simulink model "PubIfDecisionTOS_MDL"  (R2020b)
settings: configuration reference "DspaceConfig" (kept outside this file)
PostLoadFcn:
  | if any(exist('dsrtsu_mdlpostloadfcn', 'file') ~= 0), dsrtsu_mdlpostloadfcn('Execute', bdroot); end
InitFcn:
  | , if any(exist('dsmpb_private', 'file') ~= 0), dsmpb_private('dsmpb_mdlclblib', 'Init', bdroot); end,
undefined symbols (not defined in the file or in its folder): C_TOS_ACCEgoRAxletoFbumplength_m, C_TOS_ACCTargetFront_Flag, C_TOS_AEBJAPedObjDxThre_Val, C_TOS_AEBJAPedObjDyThre_Val, C_TOS_AEBJATargetSize_Val, C_TOS_AEBJAVehObjDxThre_Val, C_TOS_AEBJAVehObjDyThre_Val, C_TOS_AEBJuncPedTargetSize_Val, C_TOS_AEBLatObjDxThre_Val, C_TOS_AEBLatPedDyThre_Val, C_TOS_AEBLatTargetSize_Val, C_TOS_AEBLongTargetInEgoFront_Flag, C_TOS_axAbsGround_Parameter, C_TOS_CameraConfirmedFlag, C_TOS_CNsubjWidth, C_TOS_CurrentLaneCoreMinWidth_Val, C_TOS_CutInProb_Val_Zero, C_TOS_CutOutProb_Val_Zero, C_TOS_D2R_Val, C_TOS_DefaultValueObjectToCenterLine_dy, C_TOS_EgoCarWidth_Val, C_TOS_EgoDxRefPoint_m, C_TOS_EgoRAxletoFbumplength_m, C_TOS_HalfWidthVehicle_Con, C_TOS_HWA_CurrentLaneFlag, C_TOS_HWA_LeftLaneFlag, C_TOS_HWA_MovingDir_Vaild, C_TOS_HWA_MovState_Vaild, C_TOS_HWA_RightLaneFlag, C_TOS_LaneLineCourseErrorFront, C_TOS_LaneLineCourseErrorRear, C_TOS_MotorbikeDefaultWidth_m, C_TOS_NumberOfEffectiveTargets, C_TOS_Obj_Age_Val, C_TOS_Objdx_Constraint_Val, C_TOS_ObjectDefaultWidth_m, C_TOS_ObjInCurrentLane_Val, C_TOS_ObjInCurrentLaneValid, C_TOS_ObjInLeftLaneValid, C_TOS_ObjInRightLaneValid, C_TOS_ObjNotInCurrentLane_Val, C_TOS_ObjNotREElementType, C_TOS_ObjPredictDis_dy_ConstantVal_Zeros, C_TOS_ObjToCenterLine_ConstantVal_Zeros, C_TOS_OFMObjIDInvilad_Val, C_TOS_PIL_LatDisCons_Val_zero, C_TOS_PIL_ObjectCutInFlag_b, C_TOS_PIL_ObjectCutOutFlag_b, C_TOS_PIL_ObjLaneProb_al_Val, C_TOS_PP_ObjFusType_FC_Confirm_b, C_TOS_PP_ObjFusType_FC_FR_Confirm_b, C_TOS_PP_ObjFusType_FR_Confirm_b, C_TOS_RE_80BoolDefault_Val, C_TOS_RE_80Single181Default_Val, C_TOS_RE_80Single255Default_Val, C_TOS_RE_80Uint8Default_Val, C_TOS_RE_D2R, C_TOS_RE_D_180_Val, C_TOS_RE_InvalidObjectID_Val, C_TOS_RE_InvalidTargetChainDir_Val ... (+142)
libraries: simulink x1650, TOS_LIB x361, canfdmsglib x14
(part 10 of 69)

== system PubIfDecisionTOS_MDL/TOS_20201112/TOS_2012080320/PIL_1029/ProbCalculat/ProbFilt/ObjinLeftLaneProb ==
  PIL_ObjinLeftLaneProb : Inport
  Demux : Demux  Outputs=80
  Mux : Mux  Inputs=80
  Prob_Filt{1..80} (80 alike) : TOS_LIB/Prob_Filt  SystemSampleTime=-1  VariantActivationTime=update diagram  Latency=0  AutoFrameSizeCalculation=off
  PIL_ObjinLeftLaneProb_Filt : Outport
  wires:
  PIL_ObjinLeftLaneProb/1 -> Demux/1
  Demux/1 -> Prob_Filt1/1
  Demux/80 -> Prob_Filt72/1
  Demux/79 -> Prob_Filt71/1
  Demux/78 -> Prob_Filt70/1
  Demux/77 -> Prob_Filt69/1
  Demux/76 -> Prob_Filt68/1
  Demux/75 -> Prob_Filt67/1
  Demux/74 -> Prob_Filt66/1
  Demux/73 -> Prob_Filt80/1
  Demux/72 -> Prob_Filt79/1
  Demux/71 -> Prob_Filt78/1
  Demux/70 -> Prob_Filt77/1
  Demux/69 -> Prob_Filt76/1
  Demux/68 -> Prob_Filt75/1
  Demux/61 -> Prob_Filt46/1
  Demux/2 -> Prob_Filt2/1
  Demux/3 -> Prob_Filt3/1
  Demux/4 -> Prob_Filt4/1
  Demux/5 -> Prob_Filt5/1
  Demux/6 -> Prob_Filt6/1
  Demux/7 -> Prob_Filt7/1
  Demux/8 -> Prob_Filt8/1
  Demux/9 -> Prob_Filt9/1
  Demux/10 -> Prob_Filt10/1
  Demux/11 -> Prob_Filt11/1
  Demux/12 -> Prob_Filt12/1
  Demux/13 -> Prob_Filt13/1
  Demux/14 -> Prob_Filt14/1
  Demux/15 -> Prob_Filt15/1
  Demux/16 -> Prob_Filt16/1
  Demux/17 -> Prob_Filt17/1
  Demux/18 -> Prob_Filt25/1
  Demux/19 -> Prob_Filt26/1
  Demux/20 -> Prob_Filt27/1
  Demux/21 -> Prob_Filt28/1
  Demux/22 -> Prob_Filt29/1
  Demux/23 -> Prob_Filt30/1
  Demux/24 -> Prob_Filt31/1
  Demux/25 -> Prob_Filt32/1
  Demux/26 -> Prob_Filt18/1
  Demux/27 -> Prob_Filt19/1
  Demux/28 -> Prob_Filt20/1
  Demux/29 -> Prob_Filt21/1
  Demux/30 -> Prob_Filt22/1
  Demux/31 -> Prob_Filt23/1
  Demux/32 -> Prob_Filt24/1
  Demux/33 -> Prob_Filt33/1
  Demux/34 -> Prob_Filt44/1
  Demux/35 -> Prob_Filt55/1
  Demux/36 -> Prob_Filt59/1
  Demux/37 -> Prob_Filt60/1
  Demux/38 -> Prob_Filt61/1
  Demux/39 -> Prob_Filt62/1
  Demux/40 -> Prob_Filt63/1
  Demux/41 -> Prob_Filt64/1
  Demux/42 -> Prob_Filt34/1
  Demux/43 -> Prob_Filt35/1
  Demux/44 -> Prob_Filt36/1
  Demux/45 -> Prob_Filt37/1
  Demux/46 -> Prob_Filt38/1
  Demux/47 -> Prob_Filt39/1
  Demux/48 -> Prob_Filt40/1
  Demux/49 -> Prob_Filt41/1
  Demux/50 -> Prob_Filt50/1
  Demux/51 -> Prob_Filt51/1
  Demux/52 -> Prob_Filt52/1
  Demux/53 -> Prob_Filt53/1
  Demux/54 -> Prob_Filt54/1
  Demux/55 -> Prob_Filt56/1
  Demux/56 -> Prob_Filt57/1
  Demux/57 -> Prob_Filt58/1
  Demux/58 -> Prob_Filt42/1
  Demux/59 -> Prob_Filt43/1
  Demux/60 -> Prob_Filt45/1
  Demux/62 -> Prob_Filt47/1
  Demux/63 -> Prob_Filt48/1
  Demux/64 -> Prob_Filt49/1
  Demux/65 -> Prob_Filt65/1
  Demux/66 -> Prob_Filt73/1
  Demux/67 -> Prob_Filt74/1
  Prob_Filt1/1 -> Mux/1  "EgoCar_LeftLaneProb"
  Prob_Filt2/1 -> Mux/2  "EgoCar_LeftLaneProb"
  Prob_Filt3/1 -> Mux/3  "EgoCar_LeftLaneProb"
  Prob_Filt4/1 -> Mux/4  "EgoCar_LeftLaneProb"
  Prob_Filt5/1 -> Mux/5  "EgoCar_LeftLaneProb"
  Prob_Filt6/1 -> Mux/6  "EgoCar_LeftLaneProb"
  Prob_Filt7/1 -> Mux/7  "EgoCar_LeftLaneProb"
  Prob_Filt8/1 -> Mux/8  "EgoCar_LeftLaneProb"
  Prob_Filt9/1 -> Mux/9  "EgoCar_LeftLaneProb"
  Prob_Filt10/1 -> Mux/10  "EgoCar_LeftLaneProb"
  Prob_Filt11/1 -> Mux/11  "EgoCar_LeftLaneProb"
  Prob_Filt12/1 -> Mux/12  "EgoCar_LeftLaneProb"
  Prob_Filt13/1 -> Mux/13  "EgoCar_LeftLaneProb"
  Prob_Filt14/1 -> Mux/14  "EgoCar_LeftLaneProb"
  Prob_Filt15/1 -> Mux/15  "EgoCar_LeftLaneProb"
  Prob_Filt16/1 -> Mux/16  "EgoCar_LeftLaneProb"
  Prob_Filt17/1 -> Mux/17  "EgoCar_LeftLaneProb"
  Prob_Filt25/1 -> Mux/18  "EgoCar_LeftLaneProb"
  Prob_Filt26/1 -> Mux/19  "EgoCar_LeftLaneProb"
  Prob_Filt27/1 -> Mux/20  "EgoCar_LeftLaneProb"
  Prob_Filt28/1 -> Mux/21  "EgoCar_LeftLaneProb"
  Prob_Filt29/1 -> Mux/22  "EgoCar_LeftLaneProb"
  Prob_Filt30/1 -> Mux/23  "EgoCar_LeftLaneProb"
  Prob_Filt31/1 -> Mux/24  "EgoCar_LeftLaneProb"
  Prob_Filt32/1 -> Mux/25  "EgoCar_LeftLaneProb"
  Prob_Filt18/1 -> Mux/26  "EgoCar_LeftLaneProb"
  Prob_Filt19/1 -> Mux/27  "EgoCar_LeftLaneProb"
  Prob_Filt20/1 -> Mux/28  "EgoCar_LeftLaneProb"
  Prob_Filt21/1 -> Mux/29  "EgoCar_LeftLaneProb"
  Prob_Filt22/1 -> Mux/30  "EgoCar_LeftLaneProb"
  Prob_Filt23/1 -> Mux/31  "EgoCar_LeftLaneProb"
  Prob_Filt24/1 -> Mux/32  "EgoCar_LeftLaneProb"
  Prob_Filt33/1 -> Mux/33  "EgoCar_LeftLaneProb"
  Prob_Filt44/1 -> Mux/34  "EgoCar_LeftLaneProb"
  Prob_Filt55/1 -> Mux/35  "EgoCar_LeftLaneProb"
  Prob_Filt59/1 -> Mux/36  "EgoCar_LeftLaneProb"
  Prob_Filt60/1 -> Mux/37  "EgoCar_LeftLaneProb"
  Prob_Filt61/1 -> Mux/38  "EgoCar_LeftLaneProb"
  Prob_Filt62/1 -> Mux/39  "EgoCar_LeftLaneProb"
  Prob_Filt63/1 -> Mux/40  "EgoCar_LeftLaneProb"
  Prob_Filt64/1 -> Mux/41  "EgoCar_LeftLaneProb"
  Prob_Filt34/1 -> Mux/42  "EgoCar_LeftLaneProb"
  Prob_Filt35/1 -> Mux/43  "EgoCar_LeftLaneProb"
  Prob_Filt36/1 -> Mux/44  "EgoCar_LeftLaneProb"
  Prob_Filt37/1 -> Mux/45  "EgoCar_LeftLaneProb"
  Prob_Filt38/1 -> Mux/46  "EgoCar_LeftLaneProb"
  Prob_Filt39/1 -> Mux/47  "EgoCar_LeftLaneProb"
  Prob_Filt40/1 -> Mux/48  "EgoCar_LeftLaneProb"
  Prob_Filt41/1 -> Mux/49  "EgoCar_LeftLaneProb"
  Prob_Filt50/1 -> Mux/50  "EgoCar_LeftLaneProb"
  Prob_Filt51/1 -> Mux/51  "EgoCar_LeftLaneProb"
  Prob_Filt52/1 -> Mux/52  "EgoCar_LeftLaneProb"
  Prob_Filt53/1 -> Mux/53  "EgoCar_LeftLaneProb"
  Prob_Filt54/1 -> Mux/54  "EgoCar_LeftLaneProb"
  Prob_Filt56/1 -> Mux/55  "EgoCar_LeftLaneProb"
  Prob_Filt57/1 -> Mux/56  "EgoCar_LeftLaneProb"
  Prob_Filt58/1 -> Mux/57  "EgoCar_LeftLaneProb"
  Prob_Filt42/1 -> Mux/58  "EgoCar_LeftLaneProb"
  Prob_Filt43/1 -> Mux/59  "EgoCar_LeftLaneProb"
  Prob_Filt45/1 -> Mux/60  "EgoCar_LeftLaneProb"
  Prob_Filt46/1 -> Mux/61  "EgoCar_LeftLaneProb"
  Prob_Filt47/1 -> Mux/62  "EgoCar_LeftLaneProb"
  Prob_Filt48/1 -> Mux/63  "EgoCar_LeftLaneProb"
  Prob_Filt49/1 -> Mux/64  "EgoCar_LeftLaneProb"
  Prob_Filt65/1 -> Mux/65  "EgoCar_LeftLaneProb"
  Prob_Filt73/1 -> Mux/66  "EgoCar_LeftLaneProb"
  Prob_Filt74/1 -> Mux/67  "EgoCar_LeftLaneProb"
  Prob_Filt75/1 -> Mux/68  "EgoCar_LeftLaneProb"
  Prob_Filt76/1 -> Mux/69  "EgoCar_LeftLaneProb"
  Prob_Filt77/1 -> Mux/70  "EgoCar_LeftLaneProb"
  Prob_Filt78/1 -> Mux/71  "EgoCar_LeftLaneProb"
  Prob_Filt79/1 -> Mux/72  "EgoCar_LeftLaneProb"
  Prob_Filt80/1 -> Mux/73  "EgoCar_LeftLaneProb"
  Prob_Filt66/1 -> Mux/74  "EgoCar_LeftLaneProb"
  Prob_Filt67/1 -> Mux/75  "EgoCar_LeftLaneProb"
  Prob_Filt68/1 -> Mux/76  "EgoCar_LeftLaneProb"
  Prob_Filt69/1 -> Mux/77  "EgoCar_LeftLaneProb"
  Prob_Filt70/1 -> Mux/78  "EgoCar_LeftLaneProb"
  Prob_Filt71/1 -> Mux/79  "EgoCar_LeftLaneProb"
  Prob_Filt72/1 -> Mux/80  "EgoCar_LeftLaneProb"
  Mux/1 -> PIL_ObjinLeftLaneProb_Filt/1

== system PubIfDecisionTOS_MDL/TOS_20201112/TOS_2012080320/PIL_1029/ProbCalculat/ProbFilt/ObjinRightLaneProb ==
  PIL_ObjinRightLaneProb : Inport
  Demux : Demux  Outputs=80
  Mux : Mux  Inputs=80
  Prob_Filt{1..80} (80 alike) : TOS_LIB/Prob_Filt  SystemSampleTime=-1  VariantActivationTime=update diagram  Latency=0  AutoFrameSizeCalculation=off
  PIL_ObjinRightLaneProb_Filt : Outport
  wires:
  PIL_ObjinRightLaneProb/1 -> Demux/1
  Demux/1 -> Prob_Filt1/1
  Demux/80 -> Prob_Filt72/1
  Demux/79 -> Prob_Filt71/1
  Demux/78 -> Prob_Filt70/1
  Demux/77 -> Prob_Filt69/1
  Demux/76 -> Prob_Filt68/1
  Demux/75 -> Prob_Filt67/1
  Demux/74 -> Prob_Filt66/1
  Demux/73 -> Prob_Filt80/1
  Demux/72 -> Prob_Filt79/1
  Demux/71 -> Prob_Filt78/1
  Demux/70 -> Prob_Filt77/1
  Demux/69 -> Prob_Filt76/1
  Demux/68 -> Prob_Filt75/1
  Demux/61 -> Prob_Filt46/1
  Demux/2 -> Prob_Filt2/1
  Demux/3 -> Prob_Filt3/1
  Demux/4 -> Prob_Filt4/1
  Demux/5 -> Prob_Filt5/1
  Demux/6 -> Prob_Filt6/1
  Demux/7 -> Prob_Filt7/1
  Demux/8 -> Prob_Filt8/1
  Demux/9 -> Prob_Filt9/1
  Demux/10 -> Prob_Filt10/1
  Demux/11 -> Prob_Filt11/1
  Demux/12 -> Prob_Filt12/1
  Demux/13 -> Prob_Filt13/1
  Demux/14 -> Prob_Filt14/1
  Demux/15 -> Prob_Filt15/1
  Demux/16 -> Prob_Filt16/1
  Demux/17 -> Prob_Filt17/1
  Demux/18 -> Prob_Filt25/1
  Demux/19 -> Prob_Filt26/1
  Demux/20 -> Prob_Filt27/1
  Demux/21 -> Prob_Filt28/1
  Demux/22 -> Prob_Filt29/1
  Demux/23 -> Prob_Filt30/1
  Demux/24 -> Prob_Filt31/1
  Demux/25 -> Prob_Filt32/1
  Demux/26 -> Prob_Filt18/1
  Demux/27 -> Prob_Filt19/1
  Demux/28 -> Prob_Filt20/1
  Demux/29 -> Prob_Filt21/1
  Demux/30 -> Prob_Filt22/1
  Demux/31 -> Prob_Filt23/1
  Demux/32 -> Prob_Filt24/1
  Demux/33 -> Prob_Filt33/1
  Demux/34 -> Prob_Filt44/1
  Demux/35 -> Prob_Filt55/1
  Demux/36 -> Prob_Filt59/1
  Demux/37 -> Prob_Filt60/1
  Demux/38 -> Prob_Filt61/1
  Demux/39 -> Prob_Filt62/1
  Demux/40 -> Prob_Filt63/1
  Demux/41 -> Prob_Filt64/1
  Demux/42 -> Prob_Filt34/1
  Demux/43 -> Prob_Filt35/1
  Demux/44 -> Prob_Filt36/1
  Demux/45 -> Prob_Filt37/1
  Demux/46 -> Prob_Filt38/1
  Demux/47 -> Prob_Filt39/1
  Demux/48 -> Prob_Filt40/1
  Demux/49 -> Prob_Filt41/1
  Demux/50 -> Prob_Filt50/1
  Demux/51 -> Prob_Filt51/1
  Demux/52 -> Prob_Filt52/1
  Demux/53 -> Prob_Filt53/1
  Demux/54 -> Prob_Filt54/1
  Demux/55 -> Prob_Filt56/1
  Demux/56 -> Prob_Filt57/1
  Demux/57 -> Prob_Filt58/1
  Demux/58 -> Prob_Filt42/1
  Demux/59 -> Prob_Filt43/1
  Demux/60 -> Prob_Filt45/1
  Demux/62 -> Prob_Filt47/1
  Demux/63 -> Prob_Filt48/1
  Demux/64 -> Prob_Filt49/1
  Demux/65 -> Prob_Filt65/1
  Demux/66 -> Prob_Filt73/1
  Demux/67 -> Prob_Filt74/1
  Prob_Filt1/1 -> Mux/1  "EgoCar_LeftLaneProb"
  Prob_Filt2/1 -> Mux/2  "EgoCar_LeftLaneProb"
  Prob_Filt3/1 -> Mux/3  "EgoCar_LeftLaneProb"
  Prob_Filt4/1 -> Mux/4  "EgoCar_LeftLaneProb"
  Prob_Filt5/1 -> Mux/5  "EgoCar_LeftLaneProb"
  Prob_Filt6/1 -> Mux/6  "EgoCar_LeftLaneProb"
  Prob_Filt7/1 -> Mux/7  "EgoCar_LeftLaneProb"
  Prob_Filt8/1 -> Mux/8  "EgoCar_LeftLaneProb"
  Prob_Filt9/1 -> Mux/9  "EgoCar_LeftLaneProb"
  Prob_Filt10/1 -> Mux/10  "EgoCar_LeftLaneProb"
  Prob_Filt11/1 -> Mux/11  "EgoCar_LeftLaneProb"
  Prob_Filt12/1 -> Mux/12  "EgoCar_LeftLaneProb"
  Prob_Filt13/1 -> Mux/13  "EgoCar_LeftLaneProb"
  Prob_Filt14/1 -> Mux/14  "EgoCar_LeftLaneProb"
  Prob_Filt15/1 -> Mux/15  "EgoCar_LeftLaneProb"
  Prob_Filt16/1 -> Mux/16  "EgoCar_LeftLaneProb"
  Prob_Filt17/1 -> Mux/17  "EgoCar_LeftLaneProb"
  Prob_Filt25/1 -> Mux/18  "EgoCar_LeftLaneProb"
  Prob_Filt26/1 -> Mux/19  "EgoCar_LeftLaneProb"
  Prob_Filt27/1 -> Mux/20  "EgoCar_LeftLaneProb"
  Prob_Filt28/1 -> Mux/21  "EgoCar_LeftLaneProb"
  Prob_Filt29/1 -> Mux/22  "EgoCar_LeftLaneProb"
  Prob_Filt30/1 -> Mux/23  "EgoCar_LeftLaneProb"
  Prob_Filt31/1 -> Mux/24  "EgoCar_LeftLaneProb"
  Prob_Filt32/1 -> Mux/25  "EgoCar_LeftLaneProb"
  Prob_Filt18/1 -> Mux/26  "EgoCar_LeftLaneProb"
  Prob_Filt19/1 -> Mux/27  "EgoCar_LeftLaneProb"
  Prob_Filt20/1 -> Mux/28  "EgoCar_LeftLaneProb"
  Prob_Filt21/1 -> Mux/29  "EgoCar_LeftLaneProb"
  Prob_Filt22/1 -> Mux/30  "EgoCar_LeftLaneProb"
  Prob_Filt23/1 -> Mux/31  "EgoCar_LeftLaneProb"
  Prob_Filt24/1 -> Mux/32  "EgoCar_LeftLaneProb"
  Prob_Filt33/1 -> Mux/33  "EgoCar_LeftLaneProb"
  Prob_Filt44/1 -> Mux/34  "EgoCar_LeftLaneProb"
  Prob_Filt55/1 -> Mux/35  "EgoCar_LeftLaneProb"
  Prob_Filt59/1 -> Mux/36  "EgoCar_LeftLaneProb"
  Prob_Filt60/1 -> Mux/37  "EgoCar_LeftLaneProb"
  Prob_Filt61/1 -> Mux/38  "EgoCar_LeftLaneProb"
  Prob_Filt62/1 -> Mux/39  "EgoCar_LeftLaneProb"
  Prob_Filt63/1 -> Mux/40  "EgoCar_LeftLaneProb"
  Prob_Filt64/1 -> Mux/41  "EgoCar_LeftLaneProb"
  Prob_Filt34/1 -> Mux/42  "EgoCar_LeftLaneProb"
  Prob_Filt35/1 -> Mux/43  "EgoCar_LeftLaneProb"
  Prob_Filt36/1 -> Mux/44  "EgoCar_LeftLaneProb"
  Prob_Filt37/1 -> Mux/45  "EgoCar_LeftLaneProb"
  Prob_Filt38/1 -> Mux/46  "EgoCar_LeftLaneProb"
  Prob_Filt39/1 -> Mux/47  "EgoCar_LeftLaneProb"
  Prob_Filt40/1 -> Mux/48  "EgoCar_LeftLaneProb"
  Prob_Filt41/1 -> Mux/49  "EgoCar_LeftLaneProb"
  Prob_Filt50/1 -> Mux/50  "EgoCar_LeftLaneProb"
  Prob_Filt51/1 -> Mux/51  "EgoCar_LeftLaneProb"
  Prob_Filt52/1 -> Mux/52  "EgoCar_LeftLaneProb"
  Prob_Filt53/1 -> Mux/53  "EgoCar_LeftLaneProb"
  Prob_Filt54/1 -> Mux/54  "EgoCar_LeftLaneProb"
  Prob_Filt56/1 -> Mux/55  "EgoCar_LeftLaneProb"
  Prob_Filt57/1 -> Mux/56  "EgoCar_LeftLaneProb"
  Prob_Filt58/1 -> Mux/57  "EgoCar_LeftLaneProb"
  Prob_Filt42/1 -> Mux/58  "EgoCar_LeftLaneProb"
  Prob_Filt43/1 -> Mux/59  "EgoCar_LeftLaneProb"
  Prob_Filt45/1 -> Mux/60  "EgoCar_LeftLaneProb"
  Prob_Filt46/1 -> Mux/61  "EgoCar_LeftLaneProb"
  Prob_Filt47/1 -> Mux/62  "EgoCar_LeftLaneProb"
  Prob_Filt48/1 -> Mux/63  "EgoCar_LeftLaneProb"
  Prob_Filt49/1 -> Mux/64  "EgoCar_LeftLaneProb"
  Prob_Filt65/1 -> Mux/65  "EgoCar_LeftLaneProb"
  Prob_Filt73/1 -> Mux/66  "EgoCar_LeftLaneProb"
  Prob_Filt74/1 -> Mux/67  "EgoCar_LeftLaneProb"
  Prob_Filt75/1 -> Mux/68  "EgoCar_LeftLaneProb"
  Prob_Filt76/1 -> Mux/69  "EgoCar_LeftLaneProb"
  Prob_Filt77/1 -> Mux/70  "EgoCar_LeftLaneProb"
  Prob_Filt78/1 -> Mux/71  "EgoCar_LeftLaneProb"
  Prob_Filt79/1 -> Mux/72  "EgoCar_LeftLaneProb"
  Prob_Filt80/1 -> Mux/73  "EgoCar_LeftLaneProb"
  Prob_Filt66/1 -> Mux/74  "EgoCar_LeftLaneProb"
  Prob_Filt67/1 -> Mux/75  "EgoCar_LeftLaneProb"
  Prob_Filt68/1 -> Mux/76  "EgoCar_LeftLaneProb"
  Prob_Filt69/1 -> Mux/77  "EgoCar_LeftLaneProb"
  Prob_Filt70/1 -> Mux/78  "EgoCar_LeftLaneProb"
  Prob_Filt71/1 -> Mux/79  "EgoCar_LeftLaneProb"
  Prob_Filt72/1 -> Mux/80  "EgoCar_LeftLaneProb"
  Mux/1 -> PIL_ObjinRightLaneProb_Filt/1

== system PubIfDecisionTOS_MDL/TOS_20201112/TOS_2012080320/PP1128/AAT-AdditionalAttributes/PP_CenterLine_Calculat/EgoLane_CenterLine ==
  EgoLane : Inport
  Bus Creator1 : BusCreator  Inputs=6
  EgoLaneCenterLine01 : Subsystem
  EgoLaneCenterLine02 : Subsystem
  EgoLaneCenterLine03 : Subsystem
  EgoLaneCenterLine04 : Subsystem
  EgoLaneCenterLine05 : Subsystem
  EgoLaneCenterLine06 : Subsystem
  PP_EgoLane_CenterLine : Outport
  wires:
  EgoLane/1 -> EgoLaneCenterLine03/1(EgoLaneLine), EgoLaneCenterLine06/1(EgoLaneLine), EgoLaneCenterLine05/1(EgoLaneLine), EgoLaneCenterLine04/1(EgoLaneLine), EgoLaneCenterLine02/1(EgoLaneLine), EgoLaneCenterLine01/1(EgoLaneLine)
  EgoLaneCenterLine01/1(EgoLaneCenterLine01) -> Bus Creator1/1  "CenterLine01"
  EgoLaneCenterLine06/1(EgoLaneCenterLine06) -> Bus Creator1/6  "CenterLine06"
  EgoLaneCenterLine02/1(EgoLaneCenterLine02) -> Bus Creator1/2  "CenterLine02"
  EgoLaneCenterLine03/1(EgoLaneCenterLine03) -> Bus Creator1/3  "CenterLine03"
  EgoLaneCenterLine04/1(EgoLaneCenterLine04) -> Bus Creator1/4  "CenterLine04"
  EgoLaneCenterLine05/1(EgoLaneCenterLine05) -> Bus Creator1/5  "CenterLine05"
  Bus Creator1/1 -> PP_EgoLane_CenterLine/1  "PP_EgoLane_CenterLine"

== system PubIfDecisionTOS_MDL/TOS_20201112/TOS_2012080320/PP1128/AAT-AdditionalAttributes/PP_CenterLine_Calculat/LaneWidth ==
  LM_SignalVerification : Inport
  Add : Sum  Inputs=+-  OutDataTypeStr=single
  Add1 : Sum  Inputs=+-  OutDataTypeStr=single
  Add2 : Sum  Inputs=+-  OutDataTypeStr=single
  Bus Creator : BusCreator  Inputs=3
  Bus Selector1 : BusSelector  OutputSignals=TOS_LM_LL_Bus.LM_LL_Line04.pC0,TOS_LM_LR_Bus.LM_LR_Line04.pC0,TOS_LM_RL_Bus.LM_RL_Line04.pC0,TOS_LM_RR_Bus.LM_RR_Line04.pC0
  Saturation : Saturate  UpperLimit=4  LowerLimit=2.0  OutDataTypeStr=single
  Saturation1 : Saturate  UpperLimit=4  LowerLimit=2.0  OutDataTypeStr=single
  Saturation2 : Saturate  UpperLimit=4  LowerLimit=2.0  OutDataTypeStr=single
  Signal Copy{,1..3} (4 alike) : SignalConversion  OverrideOpt=off
  Subsystem : Subsystem  Commented=on
  PP_LaneWidth : Outport
  wires:
  Saturation/1 -> Bus Creator/1  "TOS_PP_LeftLaneWidth"
  LM_SignalVerification/1 -> Bus Selector1/1
  Saturation1/1 -> Bus Creator/2  "TOS_PP_CurrentLaneWidth"
  Bus Creator/1 -> PP_LaneWidth/1
  Saturation2/1 -> Bus Creator/3  "TOS_PP_RightLaneWidth"
  Bus Selector1/4 -> Signal Copy3/1  "<pC0>"
  Signal Copy/1 -> Add/1  "LM_LL_pC0"
  Signal Copy3/1 -> Add2/2  "LM_RR_pC0"
  Bus Selector1/2 -> Signal Copy1/1  "<pC0>"
  Add/1 -> Saturation/1
  Signal Copy1/1 -> Add1/1, Add/2  "LM_LR_pC0"
  Add1/1 -> Saturation1/1
  Bus Selector1/3 -> Signal Copy2/1  "<pC0>"
  Signal Copy2/1 -> Add1/2, Add2/1  "LM_RL_pC0"
  Add2/1 -> Saturation2/1
  Bus Selector1/1 -> Signal Copy/1  "<pC0>"

== system PubIfDecisionTOS_MDL/TOS_20201112/TOS_2012080320/PP1128/AAT-AdditionalAttributes/PP_CenterLine_Calculat/LaneWidth_80 ==
  OFM_SignalVerification : Inport
  LM_SignalVerification : Inport  Port=2
  Bus Creator : BusCreator  Inputs=3
  Bus Selector : BusSelector  OutputSignals=TOS_OFMObjValid_Flag,Object_MovingState,Object_Type
  Bus Selector1 : BusSelector  OutputSignals=TOS_LM_LL_Bus.LM_LL_Line04.pC0,TOS_LM_LR_Bus.LM_LR_Line04.pC0,TOS_LM_RL_Bus.LM_RL_Line04.pC0,TOS_LM_RR_Bus.LM_RR_Line04.pC0
  LaneWidth : Subsystem
  PP_LaneWidth : Outport
  wires:
  Bus Selector1/4 -> LaneWidth/7(LM_RR_pC0)  "<pC0>"
  Bus Selector1/3 -> LaneWidth/6(LM_RL_pC0)  "<pC0>"
  Bus Selector1/2 -> LaneWidth/5(LM_LR_pC0)  "<pC0>"
  Bus Selector1/1 -> LaneWidth/4(LM_LL_pC0)  "<pC0>"
  LaneWidth/3(TOS_PP_RightLaneWidth) -> Bus Creator/3  "TOS_PP_RightLaneWidth"
  Bus Creator/1 -> PP_LaneWidth/1
  LaneWidth/1(TOS_PP_CurrentLaneWidth) -> Bus Creator/1  "TOS_PP_CurrentLaneWidth"
  LM_SignalVerification/1 -> Bus Selector1/1
  Bus Selector/2 -> LaneWidth/2(Object_MovingState)  "<Object_MovingState>"
  Bus Selector/1 -> LaneWidth/1(TOS_OFMObjValid_Flag)  "<TOS_OFMObjValid_Flag>"
  Bus Selector/3 -> LaneWidth/3(Object_Type)  "<Object_Type>"
  OFM_SignalVerification/1 -> Bus Selector/1
  LaneWidth/2(TOS_PP_LeftLaneWidth) -> Bus Creator/2  "TOS_PP_LeftLaneWidth"

== system PubIfDecisionTOS_MDL/TOS_20201112/TOS_2012080320/PP1128/AAT-AdditionalAttributes/PP_CenterLine_Calculat/LeftLane_CenterLine ==
  LeftLane : Inport
  Bus Creator1 : BusCreator  Inputs=6
  LaneCenterLine01 : Subsystem
  LaneCenterLine02 : Subsystem
  LaneCenterLine03 : Subsystem
  LaneCenterLine04 : Subsystem
  LaneCenterLine05 : Subsystem
  LaneCenterLine06 : Subsystem
  PP_LeftLane_CenterLine : Outport
  wires:
  LeftLane/1 -> LaneCenterLine01/1(LaneLine), LaneCenterLine02/1(LaneLine), LaneCenterLine03/1(LaneLine), LaneCenterLine04/1(LaneLine), LaneCenterLine05/1(LaneLine), LaneCenterLine06/1(LaneLine)
  LaneCenterLine01/1(LaneCenterLine01) -> Bus Creator1/1  "CenterLine01"
  LaneCenterLine06/1(LaneCenterLine06) -> Bus Creator1/6  "CenterLine06"
  LaneCenterLine02/1(LaneCenterLine02) -> Bus Creator1/2  "CenterLine02"
  LaneCenterLine03/1(LaneCenterLine03) -> Bus Creator1/3  "CenterLine03"
  LaneCenterLine04/1(LaneCenterLine04) -> Bus Creator1/4  "CenterLine04"
  LaneCenterLine05/1(LaneCenterLine05) -> Bus Creator1/5  "CenterLine05"
  Bus Creator1/1 -> PP_LeftLane_CenterLine/1  "PP_LeftLane_CenterLine"

== system PubIfDecisionTOS_MDL/TOS_20201112/TOS_2012080320/PP1128/AAT-AdditionalAttributes/PP_CenterLine_Calculat/RightLane_CenterLine ==
  LeftLane : Inport
  Bus Creator1 : BusCreator  Inputs=6
  LaneCenterLine01 : Subsystem
  LaneCenterLine02 : Subsystem
  LaneCenterLine03 : Subsystem
  LaneCenterLine04 : Subsystem
  LaneCenterLine05 : Subsystem
  LaneCenterLine06 : Subsystem
  PP_RightLane_CenterLine : Outport
  wires:
  LeftLane/1 -> LaneCenterLine01/1(LaneLine), LaneCenterLine02/1(LaneLine), LaneCenterLine03/1(LaneLine), LaneCenterLine04/1(LaneLine), LaneCenterLine05/1(LaneLine), LaneCenterLine06/1(LaneLine)
  LaneCenterLine01/1(LaneCenterLine01) -> Bus Creator1/1  "CenterLine01"
  LaneCenterLine06/1(LaneCenterLine06) -> Bus Creator1/6  "CenterLine06"
  LaneCenterLine02/1(LaneCenterLine02) -> Bus Creator1/2  "CenterLine02"
  LaneCenterLine03/1(LaneCenterLine03) -> Bus Creator1/3  "CenterLine03"
  LaneCenterLine04/1(LaneCenterLine04) -> Bus Creator1/4  "CenterLine04"
  LaneCenterLine05/1(LaneCenterLine05) -> Bus Creator1/5  "CenterLine05"
  Bus Creator1/1 -> PP_RightLane_CenterLine/1  "PP_RightLane_CenterLine"

== system PubIfDecisionTOS_MDL/TOS_20201112/TOS_2012080320/PP1128/AAT-AdditionalAttributes/PP_ObjFirstDxDyDetermineSignalProcessing/PP_ObjFirstDxDyDetermine ==
  Object_ID_Last : Inport
  Object_Dx_Last : Inport  Port=2
  Object_Dy_Last : Inport  Port=3
  Object_Dx : Inport  Port=4  Partition=on  PartitionDimension=1  PartitionWidth=1  PartitionOffset=0
  Object_Dy : Inport  Port=5  Partition=on  PartitionDimension=1  PartitionWidth=1  PartitionOffset=0
  Object_ID : Inport  Port=6  Partition=on  PartitionDimension=1  PartitionWidth=1  PartitionOffset=0
  TOS_OFMObjValid_Flag : Inport  Port=7  Partition=on  PartitionDimension=1  PartitionWidth=1  PartitionOffset=0
  Compare To Constant : simulink/Logic and Bit Operations/Compare To Constant  relop===  const=C_TOS_OFMObjIDInvilad_Val  OutDataTypeStr=boolean
      settings: AttributesFormatString=C_TOS_OFMObjIDInvilad_Val = 0
  For Each : ForEach  DisableCoverage=on
  If : If  IfExpression=u1 ~= 0
  Merge : Merge
  Merge1 : Merge
  Merge2 : Merge
  PP_ObjFirstDxDyDetermine : Subsystem
  PP_ObjFirstDxDyDetermineDefault : Subsystem  TreatAsAtomicUnit=on
  Object_ID_temp : Outport  ConcatenationDimension=1
  PP_ObjFirstDetect_Dx : Outport  Port=2  ConcatenationDimension=1
  PP_ObjFirstDetect_Dy : Outport  Port=3  ConcatenationDimension=1
  wires:
  If/2 -> PP_ObjFirstDxDyDetermine/Action
  Compare To Constant/1 -> If/1
  If/1 -> PP_ObjFirstDxDyDetermineDefault/Action
  Object_Dx/1 -> PP_ObjFirstDxDyDetermine/2(Object_Dx)
  Object_Dy/1 -> PP_ObjFirstDxDyDetermine/3(Object_Dy)
  Object_ID_Last/1 -> PP_ObjFirstDxDyDetermine/4(Object_ID_Last)
  Object_Dx_Last/1 -> PP_ObjFirstDxDyDetermine/5(Object_Dx_Last)
  Object_Dy_Last/1 -> PP_ObjFirstDxDyDetermine/6(Object_Dy_Last)
  Object_ID/1 -> PP_ObjFirstDxDyDetermine/1(Object_ID)
  PP_ObjFirstDxDyDetermine/1(Object_ID_temp) -> Merge/2
  PP_ObjFirstDxDyDetermine/2(PP_ObjFirstDetect_Dx) -> Merge1/2
  PP_ObjFirstDxDyDetermine/3(PP_ObjFirstDetect_Dy) -> Merge2/2
  Merge/1 -> Object_ID_temp/1
  Merge1/1 -> PP_ObjFirstDetect_Dx/1
  Merge2/1 -> PP_ObjFirstDetect_Dy/1
  PP_ObjFirstDxDyDetermineDefault/1(Object_ID_temp) -> Merge/1
  PP_ObjFirstDxDyDetermineDefault/2(PP_ObjFirstDetect_Dx) -> Merge1/1
  PP_ObjFirstDxDyDetermineDefault/3(PP_ObjFirstDetect_Dy) -> Merge2/1
  TOS_OFMObjValid_Flag/1 -> Compare To Constant/1

== system PubIfDecisionTOS_MDL/TOS_20201112/TOS_2012080320/PP1128/AAT-AdditionalAttributes/PP_ObjectToCenterLine_dy/EgoLaneCenterLine ==
  LM_SignalVerification : Inport
  Bus Creator1 : BusCreator  Inputs=6
  EgoLaneCenterLine01 : Subsystem
  EgoLaneCenterLine02 : Subsystem
  EgoLaneCenterLine03 : Subsystem
  EgoLaneCenterLine04 : Subsystem
  EgoLaneCenterLine05 : Subsystem
  EgoLaneCenterLine06 : Subsystem
  EgoLaneCenterLine : Outport
  wires:
  LM_SignalVerification/1 -> EgoLaneCenterLine03/1(EgoLaneLine), EgoLaneCenterLine06/1(EgoLaneLine), EgoLaneCenterLine05/1(EgoLaneLine), EgoLaneCenterLine04/1(EgoLaneLine), EgoLaneCenterLine02/1(EgoLaneLine), EgoLaneCenterLine01/1(EgoLaneLine)
  EgoLaneCenterLine01/1(EgoLaneCenterLine01) -> Bus Creator1/1  "CenterLine01"
  EgoLaneCenterLine06/1(EgoLaneCenterLine06) -> Bus Creator1/6  "CenterLine06"
  EgoLaneCenterLine02/1(EgoLaneCenterLine02) -> Bus Creator1/2  "CenterLine02"
  EgoLaneCenterLine03/1(EgoLaneCenterLine03) -> Bus Creator1/3  "CenterLine03"
  EgoLaneCenterLine04/1(EgoLaneCenterLine04) -> Bus Creator1/4  "CenterLine04"
  EgoLaneCenterLine05/1(EgoLaneCenterLine05) -> Bus Creator1/5  "CenterLine05"
  Bus Creator1/1 -> EgoLaneCenterLine/1  "EgoLaneCenterLine"

== system PubIfDecisionTOS_MDL/TOS_20201112/TOS_2012080320/PP1128/AAT-AdditionalAttributes/PP_ObjectToCenterLine_dy/PP_EgoVeh_Object_ToCenterLine ==
  OFM_SignalVerification : Inport
  EgoLaneCenterLine : Inport  Port=2
  Bus Selector : BusSelector  OutputSignals=CenterLine04.PC0
  Bus Selector1 : BusSelector  OutputSignals=CenterLine01.PC0,CenterLine01.PC1,CenterLine01.PC2,CenterLine01.PC3,CenterLine01.dDisStart,CenterLine01.dDisEnd,CenterLine02.PC0,CenterLine02.PC1,CenterLine02.PC2,CenterLine02.PC3,CenterLine02.dDisStart,CenterLine02.dDisEnd,CenterLine03.PC0,CenterLine03.PC1,CenterLine03.PC2,CenterLine03.PC3,CenterLine03.dDisStart,CenterLine03.dDisEnd,CenterLine04.PC0,CenterLine04.PC1,CenterLine04.PC2,CenterLine04.PC3,CenterLine04.dDisStart,CenterLine04.dDisEnd,CenterLine05.PC0,CenterLine05.PC1,CenterLine05.PC2,CenterLine05.PC3,CenterLine05.dDisStart,CenterLine05.dDisEnd,CenterLine06.PC0,CenterLine06.PC1,CenterLine06.PC2,CenterLine06.PC3,CenterLine06.dDisStart,CenterLine06.dDisEnd
  Bus Selector2 : BusSelector  OutputSignals=TOS_OFMObjValid_Flag,Object_DY,Object_DX
  EgoVehCenterLine_dy : Subsystem
  PP_ObjectToCenterLine : Subsystem
  PP_EgoVehCenterLine_dy : Outport
  PP_ObjectToCenterLine_dy : Outport  Port=2
  wires:
  PP_ObjectToCenterLine/1(PP_ObjectToCenterLine_dy) -> PP_ObjectToCenterLine_dy/1
  Bus Selector/1 -> EgoVehCenterLine_dy/1(EgoVehCenterLine_dy)  "<PC0>"
  EgoLaneCenterLine/1 -> Bus Selector1/1, Bus Selector/1
  OFM_SignalVerification/1 -> Bus Selector2/1
  Bus Selector2/1 -> PP_ObjectToCenterLine/1(TOS_OFMObjValid_Flag)  "<TOS_OFMObjValid_Flag>"
  Bus Selector2/3 -> PP_ObjectToCenterLine/3(Object_DX)  "<Object_DX>"
  Bus Selector2/2 -> PP_ObjectToCenterLine/2(Object_DY)  "<Object_DY>"
  Bus Selector1/1 -> PP_ObjectToCenterLine/4(line01_C0)  "<PC0>"
  Bus Selector1/2 -> PP_ObjectToCenterLine/5(line01_C1)  "<PC1>"
  Bus Selector1/3 -> PP_ObjectToCenterLine/6(line01_C2)  "<PC2>"
  Bus Selector1/4 -> PP_ObjectToCenterLine/7(line01_C3)  "<PC3>"
  Bus Selector1/5 -> PP_ObjectToCenterLine/8(line01_dDisStart)  "<dDisStart>"
  Bus Selector1/6 -> PP_ObjectToCenterLine/9(line01_dDisEnd)  "<dDisEnd>"
  Bus Selector1/7 -> PP_ObjectToCenterLine/10(line02_C0)  "<PC0>"
  Bus Selector1/8 -> PP_ObjectToCenterLine/11(line02_C1)  "<PC1>"
  Bus Selector1/9 -> PP_ObjectToCenterLine/12(line02_C2)  "<PC2>"
  Bus Selector1/10 -> PP_ObjectToCenterLine/13(line02_C3)  "<PC3>"
  Bus Selector1/11 -> PP_ObjectToCenterLine/14(line02_dDisStart)  "<dDisStart>"
  Bus Selector1/12 -> PP_ObjectToCenterLine/15(line02_dDisEnd)  "<dDisEnd>"
  Bus Selector1/13 -> PP_ObjectToCenterLine/16(line03_C0)  "<PC0>"
  Bus Selector1/14 -> PP_ObjectToCenterLine/17(line03_C1)  "<PC1>"
  Bus Selector1/15 -> PP_ObjectToCenterLine/18(line03_C2)  "<PC2>"
  Bus Selector1/16 -> PP_ObjectToCenterLine/19(line03_C3)  "<PC3>"
  Bus Selector1/17 -> PP_ObjectToCenterLine/20(line03_dDisStart)  "<dDisStart>"
  Bus Selector1/18 -> PP_ObjectToCenterLine/21(line03_dDisEnd)  "<dDisEnd>"
  Bus Selector1/19 -> PP_ObjectToCenterLine/22(line04_C0)  "<PC0>"
  Bus Selector1/20 -> PP_ObjectToCenterLine/23(line04_C1)  "<PC1>"
  Bus Selector1/21 -> PP_ObjectToCenterLine/24(line04_C2)  "<PC2>"
  Bus Selector1/22 -> PP_ObjectToCenterLine/25(line04_C3)  "<PC3>"
  Bus Selector1/23 -> PP_ObjectToCenterLine/26(line04_dDisStart)  "<dDisStart>"
  Bus Selector1/24 -> PP_ObjectToCenterLine/27(line04_dDisEnd)  "<dDisEnd>"
  Bus Selector1/25 -> PP_ObjectToCenterLine/28(line05_C0)  "<PC0>"
  Bus Selector1/26 -> PP_ObjectToCenterLine/29(line05_C1)  "<PC1>"
  Bus Selector1/27 -> PP_ObjectToCenterLine/30(line05_C2)  "<PC2>"
  Bus Selector1/28 -> PP_ObjectToCenterLine/31(line05_C3)  "<PC3>"
  Bus Selector1/29 -> PP_ObjectToCenterLine/32(line05_dDisStart)  "<dDisStart>"
  Bus Selector1/30 -> PP_ObjectToCenterLine/33(line05_dDisEnd)  "<dDisEnd>"
  Bus Selector1/31 -> PP_ObjectToCenterLine/34(line06_C0)  "<PC0>"
  Bus Selector1/32 -> PP_ObjectToCenterLine/35(line06_C1)  "<PC1>"
  Bus Selector1/33 -> PP_ObjectToCenterLine/36(line06_C2)  "<PC2>"
  Bus Selector1/34 -> PP_ObjectToCenterLine/37(line06_C3)  "<PC3>"
  Bus Selector1/35 -> PP_ObjectToCenterLine/38(line06_dDisStart)  "<dDisStart>"
  Bus Selector1/36 -> PP_ObjectToCenterLine/39(line06_dDisEnd)  "<dDisEnd>"
  EgoVehCenterLine_dy/1(PP_EgoVehCenterLine_dy) -> PP_EgoVehCenterLine_dy/1

== system PubIfDecisionTOS_MDL/TOS_20201112/TOS_2012080320/PP1128/AAT-AdditionalAttributes/PP_ObjectToCenterLine_dy/PP_ObjectToCenterLine_vyc ==
  vxvRefMs : Inport
  OFM_SignalVerification : Inport  Port=2
  EgoLaneCenterLine : Inport  Port=3
  Bus Selector : BusSelector  OutputSignals=TOS_OFMObjValid_Flag,Object_ID,Object_Age
  Bus Selector1 : BusSelector  OutputSignals=CenterLine04,CenterLine05,CenterLine06
  Bus Selector2 : BusSelector  OutputSignals=Object_ID,Object_DX,Object_VX,Object_VY,TOS_OFMObjValid_Flag
  Bus Selector3 : BusSelector  OutputSignals=PC2,PC1,dDisStart,dDisEnd
  Bus Selector4 : BusSelector  OutputSignals=PC2,PC1,dDisStart,dDisEnd
  Bus Selector5 : BusSelector  OutputSignals=PC2,PC1,dDisStart,dDisEnd
  Constant1 : Constant  Value=C_TOS_NumberOfEffectiveTargets  OutDataTypeStr=int32
      settings: AttributesFormatString=C_TOS_NumberOfEffectiveTargets = 80
  ObjVyc : MATLAB Function  TreatAsAtomicUnit=on
  PP_ObjectToCenterLine_vyc_Filt : Subsystem
  PP_ObjectToCenterLine_vyc : Outport
  wires:
  ObjVyc/1(ObjVyc) -> PP_ObjectToCenterLine_vyc_Filt/4(PP_ObjectToCenterLine_vyc)
  OFM_SignalVerification/1 -> [OFM_SignalVerification], Bus Selector2/1
  EgoLaneCenterLine/1 -> Bus Selector1/1
  Bus Selector1/1 -> Bus Selector3/1  "<CenterLine04>"
  Bus Selector1/2 -> Bus Selector4/1  "<CenterLine05>"
  Bus Selector1/3 -> Bus Selector5/1  "<CenterLine06>"
  Bus Selector3/1 -> ObjVyc/1(Line04_PC2)  "<PC2>"
  Bus Selector3/2 -> ObjVyc/2(Line04_PC1)  "<PC1>"
  Bus Selector3/3 -> ObjVyc/3(Line04_dDisStart)  "<dDisStart>"
  Bus Selector3/4 -> ObjVyc/4(Line04_dDisEnd)  "<dDisEnd>"
  Bus Selector4/1 -> ObjVyc/5(Line05_PC2)  "<PC2>"
  Bus Selector4/2 -> ObjVyc/6(Line05_PC1)  "<PC1>"
  Bus Selector4/3 -> ObjVyc/7(Line05_dDisStart)  "<dDisStart>"
  Bus Selector4/4 -> ObjVyc/8(Line05_dDisEnd)  "<dDisEnd>"
  Bus Selector5/1 -> ObjVyc/9(Line06_PC2)  "<PC2>"
  Bus Selector5/2 -> ObjVyc/10(Line06_PC1)  "<PC1>"
  Bus Selector5/3 -> ObjVyc/11(Line06_dDisStart)  "<dDisStart>"
  Bus Selector5/4 -> ObjVyc/12(Line06_dDisEnd)  "<dDisEnd>"
  Bus Selector2/1 -> ObjVyc/13(Obj_ID)  "<Object_ID>"
  Bus Selector2/2 -> ObjVyc/14(Obj_Dx)  "<Object_DX>"
  Bus Selector2/3 -> ObjVyc/15(Obj_VxG)  "<Object_VX>"
  Bus Selector2/4 -> ObjVyc/16(Obj_VyG)  "<Object_VY>"
  Constant1/1 -> ObjVyc/19(C_NumberOfEffectiveTargets)
  vxvRefMs/1 -> ObjVyc/18(vxvRefMs)
  Bus Selector2/5 -> ObjVyc/17(TOS_OFMObjValid_Flag)  "<TOS_OFMObjValid_Flag>"
  PP_ObjectToCenterLine_vyc_Filt/1(PP_ObjectToCenterLine_vyc_Filt) -> PP_ObjectToCenterLine_vyc/1
  [OFM_SignalVerification] -> Bus Selector/1
  Bus Selector/2 -> PP_ObjectToCenterLine_vyc_Filt/2(Object_ID)  "<Object_ID>"
  Bus Selector/3 -> PP_ObjectToCenterLine_vyc_Filt/3(Object_Age)  "<Object_Age>"
  Bus Selector/1 -> PP_ObjectToCenterLine_vyc_Filt/1(TOS_OFMObjValid_Flag)  "<TOS_OFMObjValid_Flag>"

== system PubIfDecisionTOS_MDL/TOS_20201112/TOS_2012080320/PP1128/AAT-AdditionalAttributes/PP_SignalProcessing/PP_SignalProcessing ==
  Object_MovingState : Inport
  Object_Orientation : Inport  Port=2
  Object_AX : Inport  Port=3
  axvRefMs2 : Inport  Port=4
  Object_MovingState1 : Inport  Port=5
  Object_Fus_Type : Inport  Port=6
  Object_DX : Inport  Port=7
  Action Port : ActionPort  ActionPortLabel=else
  CamareConfirmSignalProcessing : Subsystem
  MovingState_SignalProcessing : Subsystem
  ObjFusTypeConfirm : Subsystem
  ObjMovingDirSignalProcessing : Subsystem
  ObjToEgoCarFrontbump : Subsystem
  axAbsGround : Subsystem
  PP_MovingStateSignalProcessing : Outport
  PP_MovingState_AEB_SignalProcessing : Outport  Port=2
  PP_ObjMovingDirSignalProcessing : Outport  Port=3
  PP_axAbsGround : Outport  Port=4
  PP_CamareConfirmSignalProcessing : Outport  Port=5
  PP_ObjToEgoCarFrontbump : Outport  Port=6
  PP_ObjFusType_FC_FR_Confirm : Outport  Port=7
  PP_ObjFusType_FR_Confirm : Outport  Port=8
  PP_ObjFusType_FC_Confirm : Outport  Port=9
  wires:
  Object_AX/1 -> axAbsGround/1(Object_AX)
  Object_Fus_Type/1 -> [Object_Fus_Type], CamareConfirmSignalProcessing/1(Object_FusType)
  axvRefMs2/1 -> axAbsGround/2(axvRefMs2)
  MovingState_SignalProcessing/1(PP_MovingStateSignalProcessing) -> PP_MovingStateSignalProcessing/1
  Object_MovingState/1 -> MovingState_SignalProcessing/1(Object_MovingState)
  axAbsGround/1(PP_axAbsGround) -> PP_axAbsGround/1
  Object_MovingState1/1 -> axAbsGround/3(Object_MovingState)
  CamareConfirmSignalProcessing/1(PP_CamareConfirmSignalProcessing) -> PP_CamareConfirmSignalProcessing/1
  Object_Orientation/1 -> ObjMovingDirSignalProcessing/1(Object_MovingOrientation)
  ObjToEgoCarFrontbump/1(PP_ObjToEgoCarFrontbump) -> PP_ObjToEgoCarFrontbump/1
  ObjMovingDirSignalProcessing/1(PP_ObjMovingDirSignalProcessing) -> PP_ObjMovingDirSignalProcessing/1
  Object_DX/1 -> ObjToEgoCarFrontbump/1(Object_Dx)
  [Object_Fus_Type] -> ObjFusTypeConfirm/1(Object_FusType)
  ObjFusTypeConfirm/1(ObjFusType_FC_FR_Confirm) -> PP_ObjFusType_FC_FR_Confirm/1
  ObjFusTypeConfirm/2(ObjFusType_FR_Confirm) -> PP_ObjFusType_FR_Confirm/1
  ObjFusTypeConfirm/3(ObjFusType_FC_Confirm) -> PP_ObjFusType_FC_Confirm/1
  MovingState_SignalProcessing/2(PP_MovingState_AEB_SignalProcessing) -> PP_MovingState_AEB_SignalProcessing/1

== system PubIfDecisionTOS_MDL/TOS_20201112/TOS_2012080320/PP1128/AAT-AdditionalAttributes/PP_SignalProcessing/PP_SignalProcessingDefault ==
  Action Port : ActionPort  ActionPortLabel=if(u1 ~= 0)
  Constant : Constant  Value=0  OutDataTypeStr=uint8
  Constant1 : Constant  Value=0  OutDataTypeStr=uint8
  Constant2 : Constant  Value=0  OutDataTypeStr=single
  Constant{3,5..7} (4 alike) : Constant  Value=0  OutDataTypeStr=boolean
  Constant4 : Constant  Value=255  OutDataTypeStr=single
  Constant8 : Constant  Value=0  OutDataTypeStr=uint8
  PP_MovingStateSignalProcessing : Outport
  PP_MovingState_AEB_SignalProcessing : Outport  Port=2
  PP_ObjMovingDirSignalProcessing : Outport  Port=3
  PP_axAbsGround : Outport  Port=4
  PP_CamareConfirmSignalProcessing : Outport  Port=5
  PP_ObjToEgoCarFrontbump : Outport  Port=6
  PP_ObjFusType_FC_FR_Confirm : Outport  Port=7
  PP_ObjFusType_FR_Confirm : Outport  Port=8
  PP_ObjFusType_FC_Confirm : Outport  Port=9
  wires:
  Constant/1 -> PP_MovingStateSignalProcessing/1
  Constant1/1 -> PP_ObjMovingDirSignalProcessing/1
  Constant2/1 -> PP_axAbsGround/1
  Constant3/1 -> PP_CamareConfirmSignalProcessing/1
  Constant4/1 -> PP_ObjToEgoCarFrontbump/1
  Constant7/1 -> PP_ObjFusType_FC_Confirm/1
  Constant6/1 -> PP_ObjFusType_FR_Confirm/1
  Constant5/1 -> PP_ObjFusType_FC_FR_Confirm/1
  Constant8/1 -> PP_MovingState_AEB_SignalProcessing/1

== system PubIfDecisionTOS_MDL/TOS_20201112/TOS_2012080320/PP1128/AAT-AdditionalAttributes/RoadEdge/RE_2020_12_07 ==
  OFM_OBJS : Inport  BusOutputAsStruct=on
  vxvRefMs : Inport  Port=2  OutDataTypeStr=single  PortDimensions=1  BusOutputAsStruct=on
  RoadEdge_V2 : Subsystem
  RE_EdgeElementType : Outport
  RE_StationaryObjectFlag : Outport  Port=2
  RE_EgoLeftTargetChainStartIndex : Outport  Port=3
  RE_EgoRightTargetChainStartIndex : Outport  Port=4
  RE_EgoLeftEdgeGroupChainStartIndex : Outport  Port=5
  RE_EgoRightEdgeGroupChainStartIndex : Outport  Port=6
  RE_EgoLeftStationaryObjectsSortIndex : Outport  Port=7
  RE_EgoRightStationaryObjectsSortIndex : Outport  Port=8
  RE_EdgeElementID : Outport  Port=9
  wires:
  vxvRefMs/1 -> RoadEdge_V2/2(vxvRefMs)
  OFM_OBJS/1 -> RoadEdge_V2/1(OFM_Signal)  "OFM_OBJS"
  RoadEdge_V2/1(RE_EdgeElementType) -> RE_EdgeElementType/1
  RoadEdge_V2/2(RE_StationaryObjectFlag) -> RE_StationaryObjectFlag/1
  RoadEdge_V2/7(RE_EgoLeftStationaryObjectsSortIndex) -> RE_EgoLeftStationaryObjectsSortIndex/1
  RoadEdge_V2/8(RE_EgoRightStationaryObjectsSortIndex) -> RE_EgoRightStationaryObjectsSortIndex/1
  RoadEdge_V2/6(RE_EgoRightEdgeGroupChainStartIndex) -> RE_EgoRightEdgeGroupChainStartIndex/1
  RoadEdge_V2/5(RE_EgoLeftEdgeGroupChainStartIndex) -> RE_EgoLeftEdgeGroupChainStartIndex/1
  RoadEdge_V2/4(RE_EgoRightTargetChainStartIndex) -> RE_EgoRightTargetChainStartIndex/1
  RoadEdge_V2/3(RE_EgoLeftTargetChainStartIndex) -> RE_EgoLeftTargetChainStartIndex/1
  RoadEdge_V2/9(RE_EdgeElementID) -> RE_EdgeElementID/1

== system PubIfDecisionTOS_MDL/TOS_20201112/TOS_2012080320/PP1128/AAT-AdditionalAttributes/TAP_TargetPreprocessing/OFM_SignalMaping ==
  TOS_OFMObjValid_Flag : Inport
  OFMInfo : Inport  Port=2
  Bus Creator1 : BusCreator  Inputs=31
  Bus Selector : BusSelector  OutputSignals=Object_Num,Object_Fus_Type,Object_ID,Object_Type,Object_Length,Object_Width,Object_Hight,Object_HeadingAngle,Object_YawAngle,Object_MovingState,Object_Orientation,Object_DX,Object_DY,Object_VX,Object_VY,Object_Std_AX,Object_Std_AY,Object_Std_DX,Object_Std_DY,Object_Std_VX,Object_Std_VY,Object_AX,Object_AY,Object_Std_Length,Object_Std_Width,Object_Std_HeadingAngle,Object_Type_Prob,Object_ExistProb,Object_ObstacleProb,Object_Age
  Data Type Conversion : DataTypeConversion  OutDataTypeStr=uint8
  Signal Copy{,1..27,30..31} (30 alike) : SignalConversion  OverrideOpt=off
  OFM_SignalVerification : Outport
  wires:
  Data Type Conversion/1 -> Bus Creator1/1  "TOS_OFMObjValid_Flag"
  TOS_OFMObjValid_Flag/1 -> Data Type Conversion/1  "TOS_OFMObjValid_Flag"
  Signal Copy23/1 -> Bus Creator1/19  "Object_Std_DX"
  Bus Selector/25 -> Signal Copy30/1  "<Object_Std_Width>"
  Bus Creator1/1 -> OFM_SignalVerification/1
  Bus Selector/8 -> Signal Copy7/1  "<Object_HeadingAngle>"
  Signal Copy17/1 -> Bus Creator1/21  "Object_Std_VX"
  Signal Copy19/1 -> Bus Creator1/23  "Object_AX"
  Signal Copy22/1 -> Bus Creator1/18  "Object_Std_AY"
  Signal Copy/1 -> Bus Creator1/2  "Object_Num"
  Bus Selector/20 -> Signal Copy17/1  "<Object_Std_VX>"
  Signal Copy10/1 -> Bus Creator1/12  "Object_Orientation"
  Bus Selector/21 -> Signal Copy18/1  "<Object_Std_VY>"
  Signal Copy2/1 -> Bus Creator1/4  "Object_ID"
  Signal Copy11/1 -> Bus Creator1/13  "Object_DX"
  Bus Selector/29 -> Signal Copy26/1  "<Object_ObstacleProb>"
  Signal Copy20/1 -> Bus Creator1/24  "Object_AY"
  Bus Selector/9 -> Signal Copy8/1  "<Object_YawAngle>"
  Bus Selector/5 -> Signal Copy4/1  "<Object_Length>"
  Bus Selector/12 -> Signal Copy11/1  "<Object_DX>"
  Signal Copy3/1 -> Bus Creator1/5  "Object_Type"
  Signal Copy7/1 -> Bus Creator1/9  "Object_HeadingAngle"
  Bus Selector/3 -> Signal Copy2/1  "<Object_ID>"
  Signal Copy26/1 -> Bus Creator1/30  "Object_ObstacleProb"
  Bus Selector/26 -> Signal Copy31/1  "<Object_Std_HeadingAngle>"
  Bus Selector/27 -> Signal Copy24/1  "<Object_Type_Prob>"
  Signal Copy14/1 -> Bus Creator1/16  "Object_VY"
  Bus Selector/24 -> Signal Copy21/1  "<Object_Std_Length>"
  Signal Copy24/1 -> Bus Creator1/28  "Object_Type_Prob"
  Signal Copy9/1 -> Bus Creator1/11  "Object_MovingState"
  Bus Selector/30 -> Signal Copy27/1  "<Object_Age>"
  Signal Copy16/1 -> Bus Creator1/20  "Object_Std_DY"
  Bus Selector/2 -> Signal Copy1/1  "<Object_Fus_Type>"
  Signal Copy18/1 -> Bus Creator1/22  "Object_Std_VY"
  Bus Selector/4 -> Signal Copy3/1  "<Object_Type>"
  Bus Selector/1 -> Signal Copy/1  "<Object_Num>"
  Signal Copy4/1 -> Bus Creator1/6  "Object_Length"
  Bus Selector/23 -> Signal Copy20/1  "<Object_AY>"
  Bus Selector/22 -> Signal Copy19/1  "<Object_AX>"
  Bus Selector/16 -> Signal Copy15/1  "<Object_Std_AX>"
  Signal Copy13/1 -> Bus Creator1/15  "Object_VX"
  Bus Selector/17 -> Signal Copy22/1  "<Object_Std_AY>"
  Signal Copy25/1 -> Bus Creator1/29  "Object_ExistProb"
  Bus Selector/19 -> Signal Copy16/1  "<Object_Std_DY>"
  Signal Copy27/1 -> Bus Creator1/31  "Object_Age"
  Bus Selector/18 -> Signal Copy23/1  "<Object_Std_DX>"
  Signal Copy5/1 -> Bus Creator1/7  "Object_Width"
  Signal Copy30/1 -> Bus Creator1/26  "Object_Std_Width"
  OFMInfo/1 -> Bus Selector/1
  Signal Copy8/1 -> Bus Creator1/10  "Object_YawAngle"
  Bus Selector/11 -> Signal Copy10/1  "<Object_Orientation>"
  Signal Copy6/1 -> Bus Creator1/8  "Object_Hight"
  Signal Copy12/1 -> [Object_DY]
  Bus Selector/15 -> Signal Copy14/1  "<Object_VY>"
  Signal Copy15/1 -> Bus Creator1/17  "Object_Std_AX"
  Signal Copy1/1 -> Bus Creator1/3  "Object_Fus_Type"
  Bus Selector/10 -> Signal Copy9/1  "<Object_MovingState>"
  Bus Selector/28 -> Signal Copy25/1  "<Object_ExistProb>"
  Signal Copy31/1 -> Bus Creator1/27  "Object_Std_HeadingAngle"
  Bus Selector/13 -> Signal Copy12/1  "<Object_DY>"
  Bus Selector/14 -> Signal Copy13/1  "<Object_VX>"
  Signal Copy21/1 -> Bus Creator1/25  "Object_Std_Length"
  Bus Selector/7 -> Signal Copy6/1  "<Object_Hight>"
  Bus Selector/6 -> Signal Copy5/1  "<Object_Width>"
  [Object_DY_Filt] -> Bus Creator1/14  "Object_DY"
  [Object_DY] -> [Object_DY_Filt]

== system PubIfDecisionTOS_MDL/TOS_20201112/TOS_2012080320/PP1128/AAT-AdditionalAttributes/TAP_TargetPreprocessing/TargetValidConfirm ==
  OFM_Info : Inport
  Bus Selector : BusSelector  OutputSignals=Object_ID,Object_ObstacleProb,Object_ExistProb,Object_MovingState,Object_Type,Object_Age
  TOS_OFMObjValidConfirm : Subsystem
  TOS_OFMObjValid_Flag : Outport  OutDataTypeStr=boolean
  wires:
  Bus Selector/6 -> TOS_OFMObjValidConfirm/6(Object_Age)  "<Object_Age>"
  Bus Selector/5 -> TOS_OFMObjValidConfirm/5(Object_Type)  "<Object_Type>"
  Bus Selector/4 -> TOS_OFMObjValidConfirm/4(Object_MovingState)  "<Object_MovingState>"
  Bus Selector/3 -> TOS_OFMObjValidConfirm/3(Object_ExistProb)  "<Object_ExistProb>"
  Bus Selector/2 -> TOS_OFMObjValidConfirm/2(Object_ObstacleProb)  "<Object_ObstacleProb>"
  Bus Selector/1 -> TOS_OFMObjValidConfirm/1(Object_ID)  "<Object_ID>"
  OFM_Info/1 -> Bus Selector/1
  TOS_OFMObjValidConfirm/1(TOS_OFMObjValid_Flag) -> TOS_OFMObjValid_Flag/1

== system PubIfDecisionTOS_MDL/TOS_20201112/TOS_2012080320/PP1128/ISV_InputSignalVerification/LM_SignalVerif/LM_LL_Bus ==
  LM_LINE_LL : Inport
  Bus Creator2 : BusCreator  Inputs=8  OutDataTypeStr=Bus: TOS_LM_LL_Line_bus  NonVirtualBus=on
      settings: InheritFromInputs=off
  Bus Selector1 : BusSelector  OutputSignals=LM_Line01,LM_Line02,LM_Line03,LM_Line04,LM_Line05,LM_Line06,LM_Line07,LM_Line08
  LM_LL_Line01 : Subsystem
  LM_LL_Line02 : Subsystem
  LM_LL_Line03 : Subsystem
  LM_LL_Line04 : Subsystem
  LM_LL_Line05 : Subsystem
  LM_LL_Line06 : Subsystem
  LM_LL_Line07 : Subsystem
  LM_LL_Line08 : Subsystem
  LM_LL_Bus : Outport
  wires:
  LM_LL_Line07/1(LM_LL_Line07) -> Bus Creator2/7  "LM_LL_Line07"
  Bus Selector1/1 -> LM_LL_Line01/1(LM_Line01)  "<LM_Line01>"
  Bus Selector1/5 -> LM_LL_Line05/1(LM_Line05)  "<LM_Line05>"
  Bus Selector1/4 -> LM_LL_Line04/1(LM_Line04)  "<LM_Line04>"
  LM_LL_Line01/1(LM_LL_Line01) -> Bus Creator2/1  "LM_LL_Line01"
  Bus Creator2/1 -> LM_LL_Bus/1
  Bus Selector1/7 -> LM_LL_Line07/1(LM_Line07)  "<LM_Line07>"
  Bus Selector1/3 -> LM_LL_Line03/1(LM_Line03)  "<LM_Line03>"
  LM_LL_Line05/1(LM_LL_Line05) -> Bus Creator2/5  "LM_LL_Line05"
  Bus Selector1/6 -> LM_LL_Line06/1(LM_Line06)  "<LM_Line06>"
  Bus Selector1/2 -> LM_LL_Line02/1(LM_Line02)  "<LM_Line02>"
  LM_LL_Line08/1(LM_LL_Line08) -> Bus Creator2/8  "LM_LL_Line08"
  LM_LL_Line04/1(LM_LL_Line04) -> Bus Creator2/4  "LM_LL_Line04"
  LM_LL_Line06/1(LM_LL_Line06) -> Bus Creator2/6  "LM_LL_Line06"
  Bus Selector1/8 -> LM_LL_Line08/1(LM_Line08)  "<LM_Line08>"
  LM_LL_Line02/1(LM_LL_Line02) -> Bus Creator2/2  "LM_LL_Line02"
  LM_LL_Line03/1(LM_LL_Line03) -> Bus Creator2/3  "LM_LL_Line03"
  LM_LINE_LL/1 -> Bus Selector1/1

== system PubIfDecisionTOS_MDL/TOS_20201112/TOS_2012080320/PP1128/ISV_InputSignalVerification/LM_SignalVerif/LM_LR_Bus ==
  LM_LINE_LR : Inport
  Bus Creator2 : BusCreator  Inputs=8  OutDataTypeStr=Bus: TOS_LM_LR_Line_bus  NonVirtualBus=on
      settings: InheritFromInputs=off
  Bus Selector1 : BusSelector  OutputSignals=LM_Line01,LM_Line02,LM_Line03,LM_Line04,LM_Line05,LM_Line06,LM_Line07,LM_Line08
  LM_LR_Line01 : Subsystem
  LM_LR_Line02 : Subsystem
  LM_LR_Line03 : Subsystem
  LM_LR_Line04 : Subsystem
  LM_LR_Line05 : Subsystem
  LM_LR_Line06 : Subsystem
  LM_LR_Line07 : Subsystem
  LM_LR_Line08 : Subsystem
  LM_LR_Bus : Outport
  wires:
  LM_LINE_LR/1 -> Bus Selector1/1
  LM_LR_Line03/1(LM_LR_Line03) -> Bus Creator2/3  "LM_LR_Line03"
  LM_LR_Line02/1(LM_LR_Line02) -> Bus Creator2/2  "LM_LR_Line02"
  Bus Selector1/8 -> LM_LR_Line08/1(LM_Line08)  "<LM_Line08>"
  LM_LR_Line06/1(LM_LR_Line06) -> Bus Creator2/6  "LM_LR_Line06"
  LM_LR_Line04/1(LM_LR_Line04) -> Bus Creator2/4  "LM_LR_Line04"
  LM_LR_Line08/1(LM_LR_Line08) -> Bus Creator2/8  "LM_LR_Line08"
  Bus Selector1/2 -> LM_LR_Line02/1(LM_Line02)  "<LM_Line02>"
  Bus Selector1/6 -> LM_LR_Line06/1(LM_Line06)  "<LM_Line06>"
  LM_LR_Line05/1(LM_LR_Line05) -> Bus Creator2/5  "LM_LR_Line05"
  Bus Selector1/3 -> LM_LR_Line03/1(LM_Line03)  "<LM_Line03>"
  Bus Selector1/7 -> LM_LR_Line07/1(LM_Line07)  "<LM_Line07>"
  Bus Creator2/1 -> LM_LR_Bus/1
  LM_LR_Line01/1(LM_LR_Line01) -> Bus Creator2/1  "LM_LR_Line01"
  Bus Selector1/4 -> LM_LR_Line04/1(LM_Line04)  "<LM_Line04>"
  Bus Selector1/5 -> LM_LR_Line05/1(LM_Line05)  "<LM_Line05>"
  Bus Selector1/1 -> LM_LR_Line01/1(LM_Line01)  "<LM_Line01>"
  LM_LR_Line07/1(LM_LR_Line07) -> Bus Creator2/7  "LM_LR_Line07"

== system PubIfDecisionTOS_MDL/TOS_20201112/TOS_2012080320/PP1128/ISV_InputSignalVerification/LM_SignalVerif/LM_RL_Bus ==
  LM_LINE_RL : Inport
  Bus Creator2 : BusCreator  Inputs=8  OutDataTypeStr=Bus: TOS_LM_RL_Line_bus  NonVirtualBus=on
      settings: InheritFromInputs=off
  Bus Selector1 : BusSelector  OutputSignals=LM_Line01,LM_Line02,LM_Line03,LM_Line04,LM_Line05,LM_Line06,LM_Line07,LM_Line08
  LM_RL_Line01 : Subsystem
  LM_RL_Line02 : Subsystem
  LM_RL_Line03 : Subsystem
  LM_RL_Line04 : Subsystem
  LM_RL_Line05 : Subsystem
  LM_RL_Line06 : Subsystem
  LM_RL_Line07 : Subsystem
  LM_RL_Line08 : Subsystem
  LM_RL_Bus : Outport
  wires:
  LM_RL_Line07/1(LM_RL_Line07) -> Bus Creator2/7  "LM_RL_Line07"
  Bus Selector1/1 -> LM_RL_Line01/1(LM_Line01)  "<LM_Line01>"
  Bus Selector1/5 -> LM_RL_Line05/1(LM_Line05)  "<LM_Line05>"
  Bus Selector1/4 -> LM_RL_Line04/1(LM_Line04)  "<LM_Line04>"
  LM_RL_Line01/1(LM_RL_Line01) -> Bus Creator2/1  "LM_RL_Line01"
  Bus Creator2/1 -> LM_RL_Bus/1
  Bus Selector1/7 -> LM_RL_Line07/1(LM_Line07)  "<LM_Line07>"
  Bus Selector1/3 -> LM_RL_Line03/1(LM_Line03)  "<LM_Line03>"
  LM_RL_Line05/1(LM_RL_Line05) -> Bus Creator2/5  "LM_RL_Line05"
  Bus Selector1/6 -> LM_RL_Line06/1(LM_Line06)  "<LM_Line06>"
  Bus Selector1/2 -> LM_RL_Line02/1(LM_Line02)  "<LM_Line02>"
  LM_RL_Line08/1(LM_RL_Line08) -> Bus Creator2/8  "LM_RL_Line08"
  LM_RL_Line04/1(LM_RL_Line04) -> Bus Creator2/4  "LM_RL_Line04"
  LM_RL_Line06/1(LM_RL_Line06) -> Bus Creator2/6  "LM_RL_Line06"
  Bus Selector1/8 -> LM_RL_Line08/1(LM_Line08)  "<LM_Line08>"
  LM_RL_Line02/1(LM_RL_Line02) -> Bus Creator2/2  "LM_RL_Line02"
  LM_RL_Line03/1(LM_RL_Line03) -> Bus Creator2/3  "LM_RL_Line03"
  LM_LINE_RL/1 -> Bus Selector1/1
